simulink model "gyroscope"  (R2023b)
settings: Solver=VariableStepAuto  StartTime=0.0  StopTime=100  RelTol=1e-6  AbsTol=1e-6
values from neighbouring files (symbols this model uses):
  encoder_struct = convert_cellarray_to_struct(encoder)    [main.m]
  pnet_struct = convert_cellarray_to_struct(pnet)    [main.m]
  type = 1    [main.m]
  x0 = [0; 0; 0; 0; 50; 0; 0; 0]    [main.m]
undefined symbols (not defined in the file or in its folder): fv1, fv2, fv3, fv4, i2_norm_coeff, Ib, Ic, Id, Jb, Jc, Jd, Ka, Kb, Kc, Km1, Km2, Km3, Km4, q1dot_norm_coeff, q4dot_norm_coeff, sigbuilder_block, sys_m, Ts
libraries: lpvcoreLibraryCore x8, simulink x3, vrlib x1
settings Model: NumberOfSteps=21  Creator=frank  LastModifiedBy=frank
settings DebuggingCC: AlgebraicLoopMsg=none

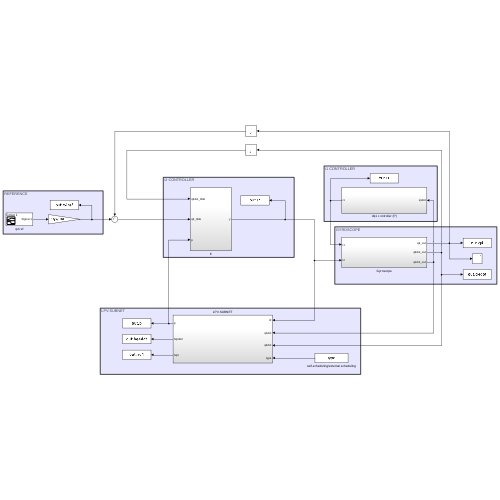
[thumbnail: Simulink's stored preview of the top-level diagram]
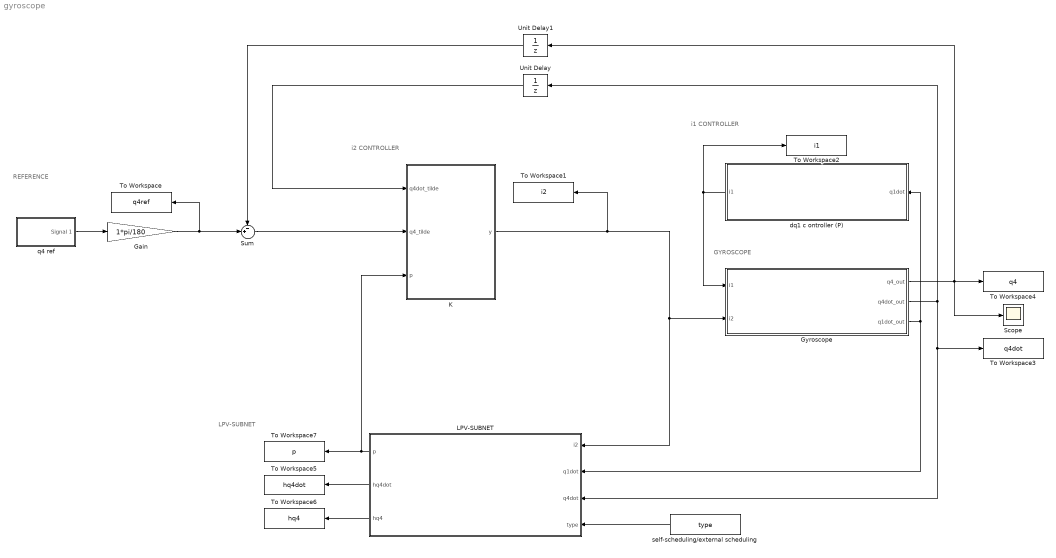
== system gyroscope ==
  note: i1 CONTROLLER
  note: REFERENCE
  note: LPV-SUBNET
  note: GYROSCOPE
  note: i2 CONTROLLER
  Gain : Gain  Gain=1*pi/180
  Gyroscope : Subsystem
  K : Subsystem
  LPV-SUBNET : Subsystem
  Scope : Scope
  Sum : Sum  Inputs=-+|
  To Workspace : ToWorkspace  VariableName=q4ref  SaveFormat=Timeseries  SampleTime=-1
  To Workspace1 : ToWorkspace  VariableName=i2  SaveFormat=Timeseries  SampleTime=-1
  To Workspace2 : ToWorkspace  VariableName=i1  SaveFormat=Timeseries  SampleTime=-1
  To Workspace3 : ToWorkspace  VariableName=q4dot  SaveFormat=Timeseries  SampleTime=-1
  To Workspace4 : ToWorkspace  VariableName=q4  SaveFormat=Timeseries  SampleTime=-1
  To Workspace5 : ToWorkspace  VariableName=hq4dot  SaveFormat=Timeseries  SampleTime=-1
  To Workspace6 : ToWorkspace  VariableName=hq4  SaveFormat=Timeseries  SampleTime=-1
  To Workspace7 : ToWorkspace  VariableName=p  SaveFormat=Timeseries  SampleTime=-1
  Unit Delay : UnitDelay  SampleTime=Ts  HasFrameUpgradeWarning=on
  Unit Delay1 : UnitDelay  SampleTime=Ts  HasFrameUpgradeWarning=on
  dq1 c ontroller (P) : Subsystem
  q4 ref : Subsystem  Tag=STV Subsys  LoadFcn=sigbuilder_block('load');  StartFcn=sigbuilder_block('start');  StopFcn=sigbuilder_block('stop');  ClipboardFcn=sigbuilder_block('clipboard');  mask(Sigbuilder block){tuvar=[0:10]}
      mask help: Simulink:masks:SigbuilderBlock_MD
      mask init:
      | if ~strcmp(get_param(bdroot(gcbh),'SimulationStatus'),'stopped') tuvar = sigbuilder_block('maskInit'); end
      settings: CopyFcn=sigbuilder_block('copy');  DeleteFcn=sigbuilder_block('delete');  ModelCloseFcn=sigbuilder_block('modelClose');  PreSaveFcn=sigbuilder_block('preSave');  PauseFcn=sigbuilder_block('pause');  ContinueFcn=sigbuilder_block('continue');  NameChangeFcn=sigbuilder_block('namechange');  OpenFcn=sigbuilder_block('open',[517.5 223.5 557.25 363 ]);  CloseFcn=sigbuilder_block('close');
      mask Display: plot(0, 0, 100, 100,[2, 2, 32, 32, 2], [68, 8, 8, 68, 68],[32, 2], [38, 38], [32, 19, 2],[53, 60, 44], [32, 17, 17, 2],[16, 16, 31, 31]);txt = getActiveGroup(gcbh);text(2, 100, txt,'verticalAlignment', 'top');
  self-scheduling/external scheduling : Constant  Value=type
  wires:
  Sum/1 -> K/2(q4_tilde)
  Gyroscope/2(q4dot_out) -> Unit Delay/1, LPV-SUBNET/3(q4dot), To Workspace3/1
  Unit Delay/1 -> K/1(q4dot_tilde)
  Gyroscope/1(q4_out) -> Scope/1, Unit Delay1/1, To Workspace4/1
  LPV-SUBNET/2(hq4dot) -> To Workspace5/1
  LPV-SUBNET/3(hq4) -> To Workspace6/1
  self-scheduling/external scheduling/1 -> LPV-SUBNET/4(type)
  LPV-SUBNET/1(p) -> To Workspace7/1, K/3(p)
  Gain/1 -> To Workspace/1, Sum/2
  dq1 c ontroller (P)/1(i1) -> Gyroscope/1(i1), To Workspace2/1
  Gyroscope/3(q1dot_out) -> LPV-SUBNET/2(q1dot), dq1 c ontroller (P)/1(q1dot)
  Unit Delay1/1 -> Sum/1
  K/1(y) -> To Workspace1/1, Gyroscope/2(i2), LPV-SUBNET/1(i2)
  q4 ref/1(Signal 1) -> Gain/1

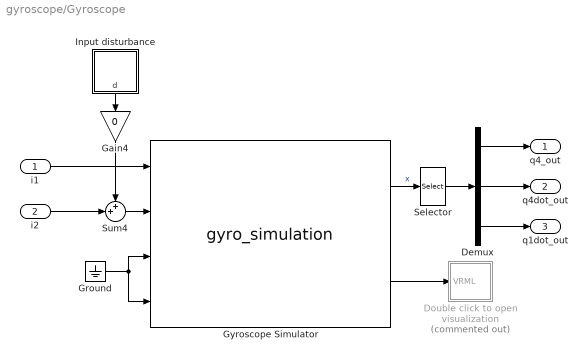
== system gyroscope/Gyroscope ==
  i1 : Inport
  i2 : Inport  Port=2
  Demux : Demux  Outputs=3
  Double click to open visualization : Subsystem  Commented=on
      settings: OpenFcn=open_system([strcat(gcb),'/Gyroscope Visualisation (open for visualisation)'],'OpenFcn')
  Gain4 : Gain  Gain=0
  Ground : Ground
  Gyroscope Simulator : S-Function  FunctionName=gyro_simulation  Parameters=x0,f,w1l,q2l,q3l,q4l,inertia,Km  SFunctionDeploymentMode=off  EnableBusSupport=off  mask(Gyroscope Simulator){x0=x0, f=[fv1;fv2;fv3;fv4], inertia=[Ib;Ic;Id;Jb;Jc;Jd;Ka;Kb;Kc], Km=[Km1;Km2;Km3;Km4], w1l=off, q2l=off, q3l=on, q4l=off}
      mask prompts: x0 "Initial conditions (x0):"; f "Viscous friction vector:"; inertia "Inertias:"; Km "Motor constants"; w1l "Disk lock"; q2l "Blue gimbal lock"; q3l "Red gimbal lock"; q4l "Silver gimbal lock"
      mask help:
      | This S-function block simulates the dynamic behavior of the gyroscope setup.
      | Click "Help" for more information.
      mask Help:
      | Outputs are the states of the gyroscope, angular positions and angular velocities, and angles for VRML simulation.
      | The outputs for the states are in the following order:
      | Position disk,
      | Position blue gimbal,
      | Position red gimbal,
      | Position silver gimbal,
      | Velocity disk,
      | Velocity blue gimbal,
      | Velocity red gimbal,
      | Velocity silver gimbal.
      | 
      | Inputs are the torques applied to the following frames:
      | Torque disk,
      | Torque blue gimbal,
      | Torque red gimbal,
      | Torque silver gimbal.
      | 
      | Parameters of the system are the initial conditions "x0" as well as lock options for each frame. The initial conditions should be entered in the same order as the state-outputs are given, seperated by a semicolon.
      | Gyroscope frames can be locked by checking the box for the corresponding frame. In case of locking, the initial conditions can be used to fix a frame under a certain angular position / velocity.
      | 
      | Viscous friction terms can be entered in a [4x1] vector in the order: [disk; blue gimbal; red gimbal; silver gimbal]
      | Inertia parameters can be entered in a [9x1] vector in the order: [Ib;Ic;Id;Jb;Jc;Jd;Ka;Kb;Kc]
      | Motor constants can be entered in a [4x1] vector in the order: [Km1;Km2;Km3;Km4]
      mask DialogControl DescGroupVar Prompt: Gyroscope Simulator
      mask DialogControl DescTextVar Prompt: Simulation block of the Quanser 3 DOF Gyroscope.
      mask DialogControl Gimbal_lock Prompt: Gimbal Lock
      mask Display:
      | disp('dx/dt = f(x,u)\n y = x')
      | image(imread('gyroscope.jpg'))
      | port_label('output',1,'States')
      | port_label('output',2,'VRML')
      | port_label('input',1,'Disk [A]')
      | port_label('input',2,'Bg [A]')
      | port_label('input',3,'Rg [A]')
      | port_label('input',4,'Sg [A]')
  Input disturbance : Subsystem
  Selector : Selector  InputPortWidth=8  IndexOptions=Index vector (dialog)  Indices=[4 8 5]  OutputSizes=1
  Sum4 : Sum  Inputs=++|
  q4_out : Outport
  q4dot_out : Outport  Port=2
  q1dot_out : Outport  Port=3
  wires:
  Demux/1 -> q4_out/1
  Gyroscope Simulator/1 -> Selector/1  "x"
  i2/1 -> Sum4/2
  Ground/1 -> Gyroscope Simulator/3, Gyroscope Simulator/4
  Gain4/1 -> Sum4/1
  Gyroscope Simulator/2 -> Double click to open visualization/1(VRML)
  i1/1 -> Gyroscope Simulator/1
  Sum4/1 -> Gyroscope Simulator/2
  Input disturbance/1(d) -> Gain4/1
  Selector/1 -> Demux/1
  Demux/2 -> q4dot_out/1
  Demux/3 -> q1dot_out/1

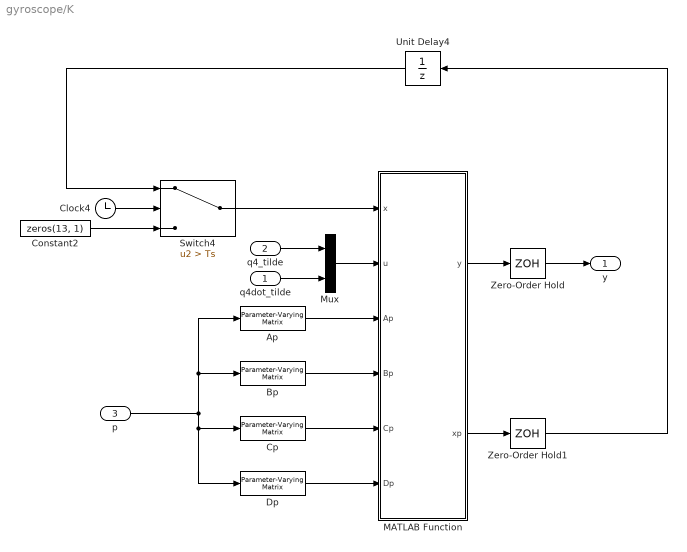
== system gyroscope/K ==
  q4dot_tilde : Inport
  q4_tilde : Inport  Port=2
  p : Inport  Port=3
  Ap : lpvcoreLibraryCore/Parameter-Varying Matrix  M=K.A
      settings: SourceProductName=LPVcore
  Bp : lpvcoreLibraryCore/Parameter-Varying Matrix  M=K.B
      settings: SourceProductName=LPVcore
  Clock4 : Clock
  Constant2 : Constant  Value=zeros(13, 1)
  Cp : lpvcoreLibraryCore/Parameter-Varying Matrix  M=K.C
      settings: SourceProductName=LPVcore
  Dp : lpvcoreLibraryCore/Parameter-Varying Matrix  M=K.D
      settings: SourceProductName=LPVcore
  MATLAB Function : MATLAB Function  TreatAsAtomicUnit=on
  Mux : Mux  Inputs=2
  Switch4 : Switch  Criteria=u2 > Threshold  Threshold=Ts  SaturateOnIntegerOverflow=off  InputSameDT=off
  Unit Delay4 : UnitDelay  SampleTime=Ts  HasFrameUpgradeWarning=on
  Zero-Order Hold : ZeroOrderHold  SampleTime=Ts
  Zero-Order Hold1 : ZeroOrderHold  SampleTime=Ts
  y : Outport
  wires:
  q4_tilde/1 -> Mux/1
  q4dot_tilde/1 -> Mux/2
  Mux/1 -> MATLAB Function/2(u)
  p/1 -> Cp/1, Dp/1, Ap/1, Bp/1
  MATLAB Function/1(y) -> Zero-Order Hold/1
  MATLAB Function/2(xp) -> Zero-Order Hold1/1
  Ap/1 -> MATLAB Function/3(Ap)
  Bp/1 -> MATLAB Function/4(Bp)
  Cp/1 -> MATLAB Function/5(Cp)
  Dp/1 -> MATLAB Function/6(Dp)
  Zero-Order Hold/1 -> y/1
  Clock4/1 -> Switch4/2
  Constant2/1 -> Switch4/3
  Switch4/1 -> MATLAB Function/1(x)
  Zero-Order Hold1/1 -> Unit Delay4/1
  Unit Delay4/1 -> Switch4/1

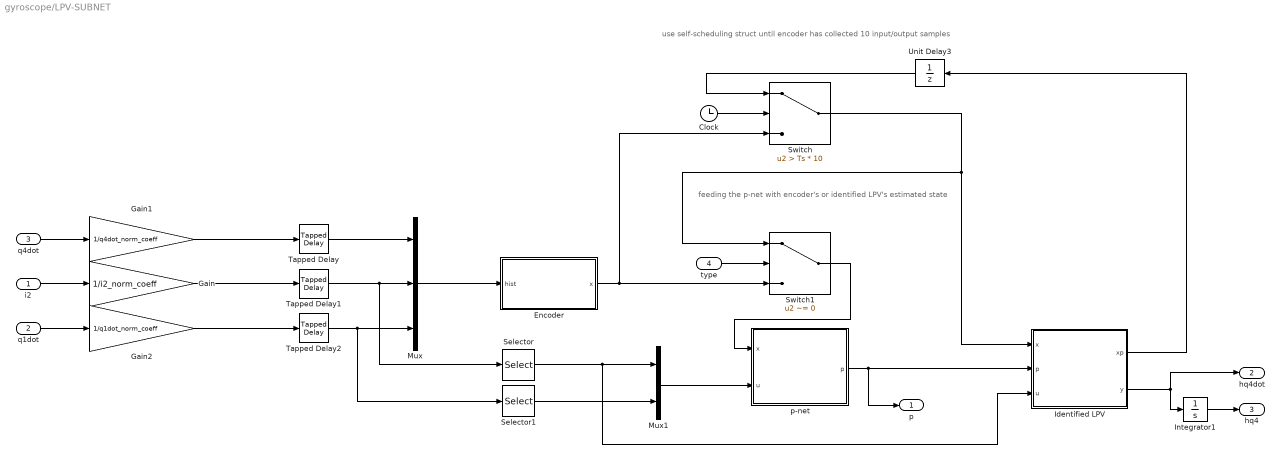
== system gyroscope/LPV-SUBNET ==
  note: feeding the p-net with encoder's or identified LPV's estimated state
  note: use self-scheduling struct until encoder has collected 10 input/output samples
  i2 : Inport
  q1dot : Inport  Port=2
  q4dot : Inport  Port=3
  type : Inport  Port=4
  Clock : Clock
  Encoder : Subsystem
  Gain : Gain  Gain=1/i2_norm_coeff
  Gain1 : Gain  Gain=1/q4dot_norm_coeff
  Gain2 : Gain  Gain=1/q1dot_norm_coeff
  Identified LPV : Subsystem
  Integrator1 : Integrator
  Mux : Mux  Inputs=3
  Mux1 : Mux  Inputs=2
  Selector : Selector  InputPortWidth=10  IndexOptions=Index vector (dialog)  Indices=1  OutputSizes=1
  Selector1 : Selector  InputPortWidth=10  IndexOptions=Index vector (dialog)  Indices=1  OutputSizes=1
  Switch : Switch  Criteria=u2 > Threshold  Threshold=Ts * 10  SaturateOnIntegerOverflow=off  InputSameDT=off
  Switch1 : Switch  Criteria=u2 ~= 0  Threshold=Ts * 10  SaturateOnIntegerOverflow=off  InputSameDT=off
  Tapped Delay : simulink/Discrete/Tapped Delay  vinit=0.0  samptime=Ts  NumDelays=10  DelayOrder=Newest  includeCurrent=off
  Tapped Delay1 : simulink/Discrete/Tapped Delay  vinit=0.0  samptime=Ts  NumDelays=10  DelayOrder=Newest  includeCurrent=off
  Tapped Delay2 : simulink/Discrete/Tapped Delay  vinit=0.0  samptime=Ts  NumDelays=10  DelayOrder=Newest  includeCurrent=off
  Unit Delay3 : UnitDelay  SampleTime=Ts  HasFrameUpgradeWarning=on
  p-net : Subsystem
  p : Outport
  hq4dot : Outport  Port=2
  hq4 : Outport  Port=3
  wires:
  Identified LPV/1(xp) -> Unit Delay3/1
  Unit Delay3/1 -> Switch/1
  Identified LPV/2(y) -> Integrator1/1, hq4dot/1
  Clock/1 -> Switch/2
  Switch/1 -> Identified LPV/1(x), Switch1/1
  Tapped Delay/1 -> Mux/1
  i2/1 -> Gain/1
  Encoder/1(x) -> Switch/3, Switch1/3
  p-net/1(p) -> Identified LPV/2(p), p/1
  Gain/1 -> Tapped Delay1/1
  q4dot/1 -> Gain1/1
  Integrator1/1 -> hq4/1
  Mux1/1 -> p-net/2(u)
  Tapped Delay2/1 -> Selector1/1, Mux/3
  type/1 -> Switch1/2
  Switch1/1 -> p-net/1(x)
  Mux/1 -> Encoder/1(hist)
  q1dot/1 -> Gain2/1
  Gain2/1 -> Tapped Delay2/1
  Tapped Delay1/1 -> Selector/1, Mux/2
  Gain1/1 -> Tapped Delay/1
  Selector/1 -> Identified LPV/3(u), Mux1/1
  Selector1/1 -> Mux1/2

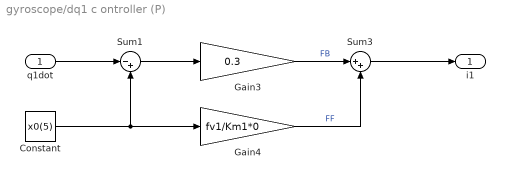
== system gyroscope/dq1 c ontroller (P) ==
  q1dot : Inport
  Constant : Constant  Value=x0(5)
  Gain3 : Gain  Gain=0.3
  Gain4 : Gain  Gain=fv1/Km1*0
  Sum1 : Sum  Inputs=|-+
  Sum3 : Sum  Inputs=|++
  i1 : Outport
  wires:
  Gain4/1 -> Sum3/2  "FF"
  Sum1/1 -> Gain3/1
  q1dot/1 -> Sum1/1
  Sum3/1 -> i1/1
  Gain3/1 -> Sum3/1  "FB"
  Constant/1 -> Sum1/2, Gain4/1

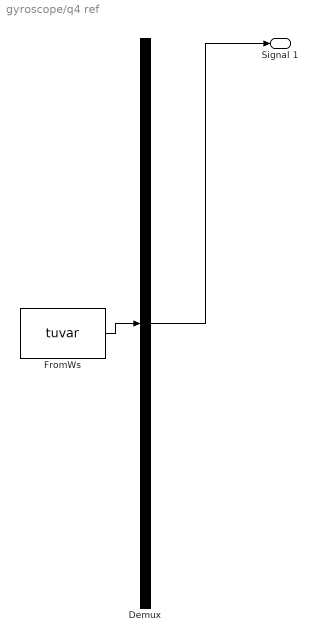
== system gyroscope/q4 ref ==
  Demux : Demux  Tag=STV Demux  Outputs=1
      settings: DisplayOption=none
  FromWs : FromWorkspace  Tag=STV FromWs  VariableName=tuvar
      SigBuilderData=|
      | common.afterFinalStr = 'Extrapolate'
      | common.sampleTime = 0
      | dataSet.timeRange = [0 50]
      | dataSet.name = 'Group 1'
      | sbobj.Groups.Name = 'Group 1'
      | sbobj.Groups.Signals.Name = 'Signal 1'
      | sbobj.Groups.Signals.XData = [0 4.9 10 10 15 20.1 20.1 30 30 50]
      | sbobj.Groups.Signals.YData = [45 45 45 0 0 0 -45 -45.5 0 0]
      | sbobj.Groups.TimeRange = [0 50]
  Signal 1 : Outport  Tag=STV Outport
  wires:
  Demux/1 -> Signal 1/1
  FromWs/1 -> Demux/1

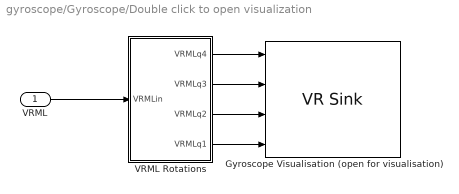
== system gyroscope/Gyroscope/Double click to open visualization ==
  VRML : Inport
  Gyroscope Visualisation (open for visualisation) : vrlib/VR Sink  InstantiateOnLoad=on  SampleTime=0.03333333  ViewEnable=on  RemoteChange=off  RemoteView=off  FieldsWritten=SG.rotation.4.1.1.double#RG.rotation.4.1.1.double#BG.rotation.4.1.1.double#Disk.rotation.4.1.1.double  WorldFileName=World/Gyroscope_Visualisation.wrl  WorldDescription=Gyroscope Visualisation  AutoView=off  VideoDimensions=[]  AllowVariableSize=off  FigureProperties=[]
  "VRML Rotations " : Subsystem
  wires:
  VRML/1 -> "VRML Rotations "/1(VRMLin)
  "VRML Rotations "/1(VRMLq4) -> Gyroscope Visualisation (open for visualisation)/1
  "VRML Rotations "/2(VRMLq3) -> Gyroscope Visualisation (open for visualisation)/2
  "VRML Rotations "/4(VRMLq1) -> Gyroscope Visualisation (open for visualisation)/4
  "VRML Rotations "/3(VRMLq2) -> Gyroscope Visualisation (open for visualisation)/3

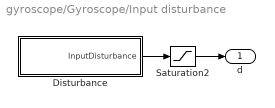
== system gyroscope/Gyroscope/Input disturbance ==
  Disturbance : Subsystem  Tag=STV Subsys  LoadFcn=sigbuilder_block('load');  StartFcn=sigbuilder_block('start');  StopFcn=sigbuilder_block('stop');  ClipboardFcn=sigbuilder_block('clipboard');  mask(Sigbuilder block){tuvar=[0:10]}
      mask help: Simulink:masks:SigbuilderBlock_MD
      mask init:
      | if ~strcmp(get_param(bdroot(gcbh),'SimulationStatus'),'stopped') tuvar = sigbuilder_block('maskInit'); end
      settings: CopyFcn=sigbuilder_block('copy');  DeleteFcn=sigbuilder_block('delete');  ModelCloseFcn=sigbuilder_block('modelClose');  PreSaveFcn=sigbuilder_block('preSave');  PauseFcn=sigbuilder_block('pause');  ContinueFcn=sigbuilder_block('continue');  NameChangeFcn=sigbuilder_block('namechange');  OpenFcn=sigbuilder_block('open',[517.5 223.5 557.25 363 ]);  CloseFcn=sigbuilder_block('close');
      mask Display: plot(0, 0, 100, 100,[2, 2, 32, 32, 2], [68, 8, 8, 68, 68],[32, 2], [38, 38], [32, 19, 2],[53, 60, 44], [32, 17, 17, 2],[16, 16, 31, 31]);txt = getActiveGroup(gcbh);text(2, 100, txt,'verticalAlignment', 'top');
  Saturation2 : Saturate  UpperLimit=0.1  LowerLimit=-0.1
  d : Outport
  wires:
  Saturation2/1 -> d/1
  Disturbance/1(InputDisturbance) -> Saturation2/1

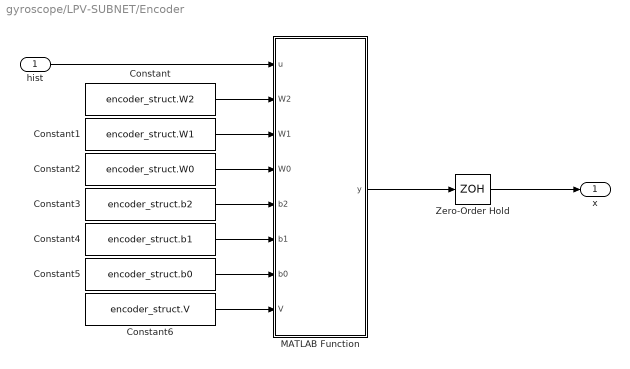
== system gyroscope/LPV-SUBNET/Encoder ==
  hist : Inport
  Constant : Constant  Value=encoder_struct.W2
  Constant1 : Constant  Value=encoder_struct.W1
  Constant2 : Constant  Value=encoder_struct.W0
  Constant3 : Constant  Value=encoder_struct.b2
  Constant4 : Constant  Value=encoder_struct.b1
  Constant5 : Constant  Value=encoder_struct.b0
  Constant6 : Constant  Value=encoder_struct.V
  MATLAB Function : MATLAB Function  TreatAsAtomicUnit=on
  Zero-Order Hold : ZeroOrderHold  SampleTime=Ts
  x : Outport
  wires:
  hist/1 -> MATLAB Function/1(u)
  Constant/1 -> MATLAB Function/2(W2)
  MATLAB Function/1(y) -> Zero-Order Hold/1
  Constant1/1 -> MATLAB Function/3(W1)
  Constant2/1 -> MATLAB Function/4(W0)
  Constant3/1 -> MATLAB Function/5(b2)
  Constant4/1 -> MATLAB Function/6(b1)
  Constant5/1 -> MATLAB Function/7(b0)
  Constant6/1 -> MATLAB Function/8(V)
  Zero-Order Hold/1 -> x/1

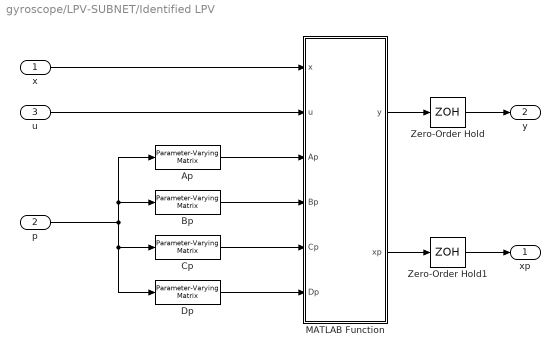
== system gyroscope/LPV-SUBNET/Identified LPV ==
  x : Inport
  p : Inport  Port=2
  u : Inport  Port=3
  Ap : lpvcoreLibraryCore/Parameter-Varying Matrix  M=sys_m{1}
      settings: SourceProductName=LPVcore
  Bp : lpvcoreLibraryCore/Parameter-Varying Matrix  M=sys_m{2}
      settings: SourceProductName=LPVcore
  Cp : lpvcoreLibraryCore/Parameter-Varying Matrix  M=sys_m{3}
      settings: SourceProductName=LPVcore
  Dp : lpvcoreLibraryCore/Parameter-Varying Matrix  M=sys_m{4}
      settings: SourceProductName=LPVcore
  MATLAB Function : MATLAB Function  TreatAsAtomicUnit=on
  Zero-Order Hold : ZeroOrderHold  SampleTime=Ts
  Zero-Order Hold1 : ZeroOrderHold  SampleTime=Ts
  xp : Outport
  y : Outport  Port=2
  wires:
  p/1 -> Dp/1, Cp/1, Ap/1, Bp/1
  MATLAB Function/1(y) -> Zero-Order Hold/1
  MATLAB Function/2(xp) -> Zero-Order Hold1/1
  x/1 -> MATLAB Function/1(x)
  u/1 -> MATLAB Function/2(u)
  Ap/1 -> MATLAB Function/3(Ap)
  Bp/1 -> MATLAB Function/4(Bp)
  Cp/1 -> MATLAB Function/5(Cp)
  Dp/1 -> MATLAB Function/6(Dp)
  Zero-Order Hold/1 -> y/1
  Zero-Order Hold1/1 -> xp/1

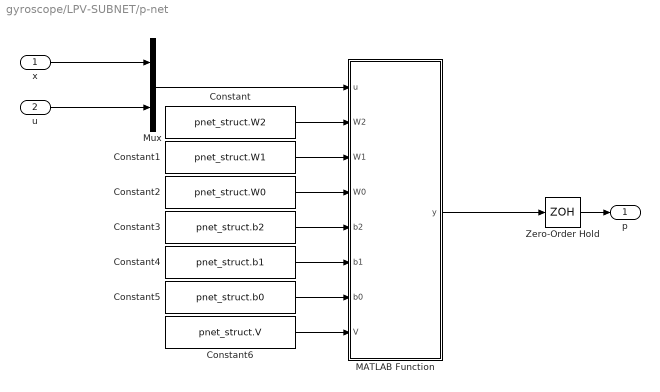
== system gyroscope/LPV-SUBNET/p-net ==
  x : Inport
  u : Inport  Port=2
  Constant : Constant  Value=pnet_struct.W2
  Constant1 : Constant  Value=pnet_struct.W1
  Constant2 : Constant  Value=pnet_struct.W0
  Constant3 : Constant  Value=pnet_struct.b2
  Constant4 : Constant  Value=pnet_struct.b1
  Constant5 : Constant  Value=pnet_struct.b0
  Constant6 : Constant  Value=pnet_struct.V
  MATLAB Function : MATLAB Function  TreatAsAtomicUnit=on
  Mux : Mux  Inputs=2
  Zero-Order Hold : ZeroOrderHold  SampleTime=Ts
  p : Outport
  wires:
  x/1 -> Mux/1
  u/1 -> Mux/2
  Mux/1 -> MATLAB Function/1(u)
  Constant1/1 -> MATLAB Function/3(W1)
  Constant3/1 -> MATLAB Function/5(b2)
  Constant6/1 -> MATLAB Function/8(V)
  Constant2/1 -> MATLAB Function/4(W0)
  Constant/1 -> MATLAB Function/2(W2)
  Constant5/1 -> MATLAB Function/7(b0)
  Constant4/1 -> MATLAB Function/6(b1)
  Zero-Order Hold/1 -> p/1
  MATLAB Function/1(y) -> Zero-Order Hold/1

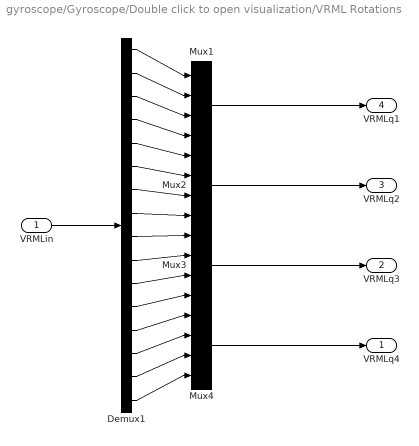
== system gyroscope/Gyroscope/Double click to open visualization/VRML Rotations  ==
  VRMLin : Inport
  Demux1 : Demux  Outputs=16
  Mux{1..4} (4 alike) : Mux
  VRMLq4 : Outport
  VRMLq3 : Outport  Port=2
  VRMLq2 : Outport  Port=3
  VRMLq1 : Outport  Port=4
  wires:
  Mux1/1 -> VRMLq1/1
  Demux1/3 -> Mux1/3
  Demux1/8 -> Mux2/4
  Demux1/14 -> Mux4/2
  Demux1/12 -> Mux3/4
  Demux1/11 -> Mux3/3
  Demux1/13 -> Mux4/1
  Demux1/16 -> Mux4/4
  Mux4/1 -> VRMLq4/1
  Demux1/9 -> Mux3/1
  Demux1/7 -> Mux2/3
  Demux1/10 -> Mux3/2
  Demux1/15 -> Mux4/3
  Mux3/1 -> VRMLq3/1
  Mux2/1 -> VRMLq2/1
  Demux1/5 -> Mux2/1
  Demux1/2 -> Mux1/2
  Demux1/4 -> Mux1/4
  Demux1/1 -> Mux1/1
  Demux1/6 -> Mux2/2
  VRMLin/1 -> Demux1/1

== system gyroscope/Gyroscope/Input disturbance/Disturbance ==
  Demux : Demux  Tag=STV Demux  Outputs=1
      settings: DisplayOption=none
  FromWs : FromWorkspace  Tag=STV FromWs  VariableName=tuvar
      SigBuilderData=|
      | common.afterFinalStr = 'Extrapolate'
      | common.sampleTime = 0
      | dataSet.timeRange = [0 50]
      | dataSet.name = 'Group 1'
      | sbobj.Groups.Name = 'Group 1'
      | sbobj.Groups.Signals.Name = 'InputDisturbance'
      | sbobj.Groups.Signals.XData = [0 0.1 0.2 0.3 0.4 0.5 0.6 0.7 0.8 0.9 1 1.1 ... (501 elements, 1x501)]
      | sbobj.Groups.Signals.YData = [-0.189723560894 0.131851962851 0.0532358984717 0.0601597721194 0.0467188654102 0.020818147654 -0.00575993913192 -0.306518570597 -0.061249415713 -0.00161618872855 0.0776899839858 -0.00900061185687 ... (501 elements, 1x501)]
      | sbobj.Groups.TimeRange = [0 50]
  InputDisturbance : Outport  Tag=STV Outport
  wires:
  Demux/1 -> InputDisturbance/1
  FromWs/1 -> Demux/1

== matlab function gyroscope/LPV-SUBNET/p-net/MATLAB Function ==
  data: u input; y output; W2 input; W1 input; W0 input; b2 input; b1 input; b0 input; V input
function y = fcn(u, W2, W1, W0, b2, b1, b0, V)

nonlin = W2 * tanh(W1 * ...
    tanh(W0 * u + b0) + b1) + b2;
y = V * u + nonlin;

== matlab function gyroscope/LPV-SUBNET/Encoder/MATLAB Function ==
  data: u input; y output; W2 input; W1 input; W0 input; b2 input; b1 input; b0 input; V input
function y = fcn(u, W2, W1, W0, b2, b1, b0, V)

nonlin = W2 * tanh(W1 * ...
    tanh(W0 * u + b0) + b1) + b2;
y = V * u + nonlin;

== matlab function gyroscope/LPV-SUBNET/Identified LPV/MATLAB Function ==
  data: x input; u input; y output; xp output; Ap input; Bp input; Cp input; Dp input
function [y, xp] = fcn(x, u, Ap, Bp, Cp, Dp)

y = Cp * x + Dp * u;
xp = Ap * x + Bp * u;

== matlab function gyroscope/K/MATLAB Function ==
  data: x input; u input; y output; xp output; Ap input; Bp input; Cp input; Dp input
function [y, xp] = fcn(x, u, Ap, Bp, Cp, Dp)

y = Cp * x + Dp * u;
xp = Ap * x + Bp * u;
